simulink model "M182_Lab0"  (R2019b)
settings: Solver=VariableStepAuto  StartTime=0.0  StopTime=30  RelTol=1e-3
settings Model: Creator=scjcb  LastModifiedBy=scjcb

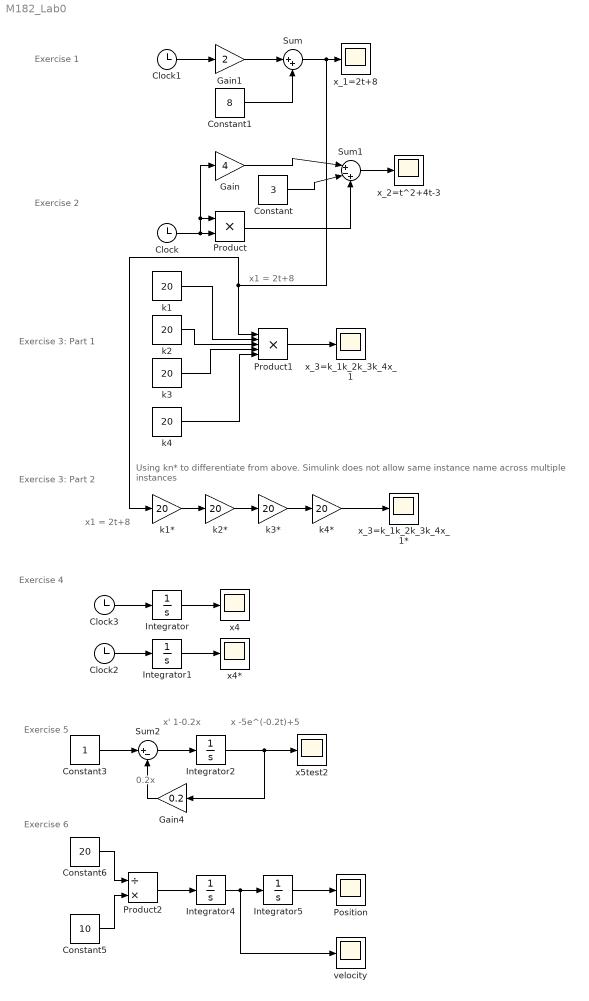
== system M182_Lab0 ==
  note: x
      | -5e^(-0.2t)+5
  note: x'
      | 1-0.2x
  note: Exercise 2
  note: Exercise 1
  note: Exercise 3: Part 1
  note: Exercise 3: Part 2
  note: Using kn* to differentiate from above. Simulink does not allow same instance name across multiple instances
  note: x1 = 2t+8
  note: x1 = 2t+8
  note: Exercise 4
  note: 0.2x
  note: Exercise 5
  note: Exercise 6
  Clock{,1..3} (4 alike) : Clock
  Constant : Constant  Value=3
  Constant1 : Constant  Value=8
  Constant3 : Constant
  Constant5 : Constant  Value=10
  Constant6 : Constant  Value=20
  Gain : Gain  Gain=4
  Gain1 : Gain  Gain=2
  Gain4 : Gain  Gain=0.2
  Integrator{,2,4..5} (4 alike) : Integrator
  Integrator1 : Integrator  InitialCondition=50
  Position : Scope
  Product : Product
  Product1 : Product  Inputs=5
  Product2 : Product  Inputs=/*
  Sum : Sum  Inputs=|++
  Sum1 : Sum  Inputs=|+-+
  Sum2 : Sum  Inputs=|+-
  k{1..4} (4 alike) : Constant  Value=20
  k1* : Gain  Gain=20
  k2* : Gain  Gain=20
  k3* : Gain  Gain=20
  k4* : Gain  Gain=20
  velocity : Scope
  x4 : Scope
  x4* : Scope
  x5test2 : Scope
  x_1=2t+8 : Scope
  x_2=t^2+4t-3 : Scope
  x_3=k_1k_2k_3k_4x_1 : Scope
  x_3=k_1k_2k_3k_4x_1* : Scope
  wires:
  Gain/1 -> Sum1/1
  Clock/1 -> Gain/1, Product/1, Product/2
  Constant/1 -> Sum1/2
  Sum1/1 -> x_2=t^2+4t-3/1
  Product/1 -> Sum1/3
  Clock1/1 -> Gain1/1
  Gain1/1 -> Sum/1
  Constant1/1 -> Sum/2
  Sum/1 -> k1*/1, Product1/1, x_1=2t+8/1
  k1/1 -> Product1/2
  k2/1 -> Product1/3
  k3/1 -> Product1/4
  k4/1 -> Product1/5
  Product1/1 -> x_3=k_1k_2k_3k_4x_1/1
  k1*/1 -> k2*/1
  k2*/1 -> k3*/1
  k3*/1 -> k4*/1
  k4*/1 -> x_3=k_1k_2k_3k_4x_1*/1
  Clock3/1 -> Integrator/1
  Integrator/1 -> x4/1
  Clock2/1 -> Integrator1/1
  Integrator1/1 -> x4*/1
  Constant3/1 -> Sum2/1
  Integrator2/1 -> x5test2/1, Gain4/1
  Gain4/1 -> Sum2/2
  Sum2/1 -> Integrator2/1
  Integrator4/1 -> velocity/1, Integrator5/1
  Integrator5/1 -> Position/1
  Constant5/1 -> Product2/2
  Constant6/1 -> Product2/1
  Product2/1 -> Integrator4/1
